simulink model "PRH_PI"  (R2021a)
settings: Solver=FixedStepDiscrete  StartTime=0.0  StopTime=4  RelTol=1e-3
values from neighbouring files (symbols this model uses):
  kp = place(A, B, [-8+.8i -8-.8i -9+.9i -9-.9i, -2+.1i, -2-.1i])    [HeightControlWithStableAngle.m]
  kr = transpose(transpose(V)*(V*transpose(V))^-1)    [HeightControlWithStableAngle.m]    (also in YawPitchRollHeightControl.m)
undefined symbols (not defined in the file or in its folder): DiscIntNeverNeededParam, Newton, Raphson
settings Model: Creator=tocay  LastModifiedBy=tocay
settings OptimizationCC: DefaultParameterBehavior=Inlined  UseDivisionForNetSlopeComputation=on  GainParamInheritBuiltInType=on  UseFloatMulNetSlope=on  InlineInvariantSignals=on  PassReuseOutputArgsAs=Individual arguments  ZeroExternalMemoryAtStartup=off  ZeroInternalMemoryAtStartup=off  NoFixptDivByZeroProtection=on  EfficientFloat2IntCast=on  LifeSpan=1  OptimizeBlockOrder=speed  DifferentSizesBufferReuse=on  EfficientTunableParamExpr=on
settings DebuggingCC: ParameterTunabilityLossMsg=error
settings HardwareCC: ProdBitPerInt=16  ProdBitPerPointer=8  ProdBitPerSizeT=24  ProdBitPerPtrDiffT=24  ProdLargestAtomicFloat=None  ProdWordSize=8  ProdLongLongMode=on  ProdHWDeviceType=Microchip->PIC18
settings SFSimCC: MATLABDynamicMemAlloc=off
settings RTWCC: SystemTargetFile=ert.tlc  GenCodeOnly=on  PackageName=PRH_at2.zip  TemplateMakefile=ert_default_tmf  TargetLang=C++
settings CodeAppCC: ForceParamTrailComments=on  IgnoreCustomStorageClasses=off  OperatorAnnotations=on  SimulinkDataObjDesc=on  SFDataObjDesc=on  CustomSymbolStrGlobalVar=rt$N$M  CustomSymbolStrType=$N$M  CustomSymbolStrFcn=$N$M$F  CustomSymbolStrMacro=$N$M  InsertBlockDesc=on
settings ERTTargetCC: TargetLangStandard=C++03 (ISO)  GenerateSampleERTMain=on  IncludeMdlTerminateFcn=off  CombineSignalStateStructs=on  SuppressErrorStatus=on  SupportAbsoluteTime=off  CodeInterfacePackaging=C++ class  SupportComplex=off  InlinedParameterPlacement=NonHierarchical  RootIOFormat=Structure reference  ERTCustomFileTemplate=example_file_process.tlc  ERTFilePackagingFormat=CompactWithDataFile

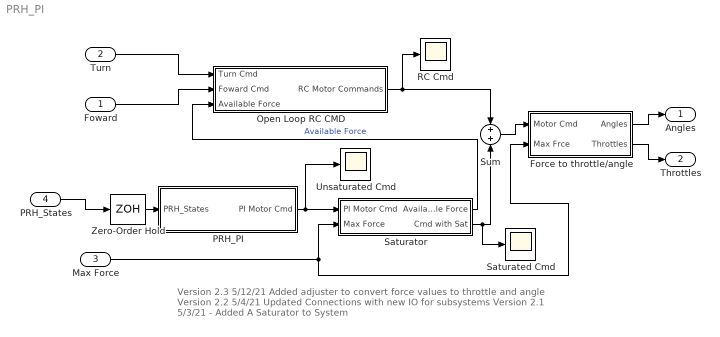
== system PRH_PI ==
  note: Version 2.3 5/12/21 Added adjuster to convert force values to throttle and angle
      | Version 2.2 5/4/21 Updated Connections with new IO for subsystems
      | Version 2.1 5/3/21 - Added A Saturator to System
  Foward : Inport
  Turn : Inport  Port=2
  Max Force : Inport  Port=3
  PRH_States : Inport  Port=4
  Force to throttle/angle : Subsystem
  Open Loop RC CMD : Subsystem
  PRH_PI : Subsystem
  RC Cmd : Scope
  Saturated Cmd : Scope
  Saturator : Subsystem
  Sum : Sum
  Unsaturated Cmd : Scope
  Zero-Order Hold : ZeroOrderHold  SampleTime=-1
  Angles : Outport
  Throttles : Outport  Port=2
  wires:
  Turn/1 -> Open Loop RC CMD/1(Turn Cmd)
  Open Loop RC CMD/1(RC Motor Commands) -> RC Cmd/1, Sum/1
  PRH_PI/1(PI Motor Cmd) -> Unsaturated Cmd/1, Saturator/1(PI Motor Cmd)
  Sum/1 -> Force to throttle/angle/1(Motor Cmd)
  Force to throttle/angle/2(Throttles) -> Throttles/1
  Force to throttle/angle/1(Angles) -> Angles/1
  Foward/1 -> Open Loop RC CMD/2(Foward Cmd)
  Saturator/1(Available Force) -> Open Loop RC CMD/3(Available Force)  "Available Force"
  Saturator/2(Cmd with Sat) -> Saturated Cmd/1, Sum/2
  Max Force/1 -> Saturator/2(Max Force), Force to throttle/angle/2(Max Frce)
  Zero-Order Hold/1 -> PRH_PI/1(PRH_States)
  PRH_States/1 -> Zero-Order Hold/1

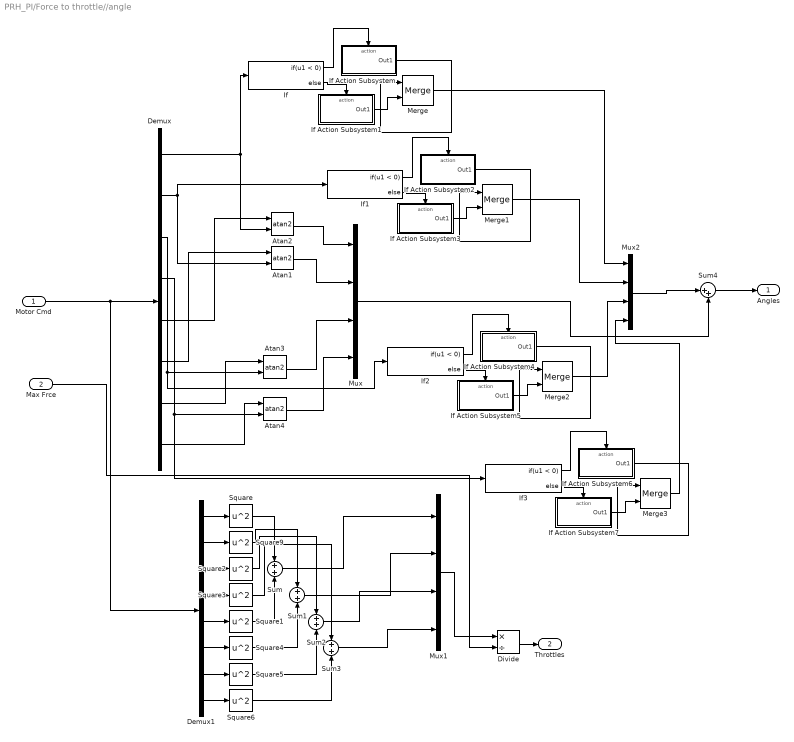
== system PRH_PI/Force to throttle//angle ==
  Motor Cmd : Inport
  Max Frce : Inport  Port=2
  Atan{1..4} (4 alike) : Trigonometry  Operator=atan2
  Demux : Demux  Outputs=8
  Demux1 : Demux  Outputs=8
  Divide : Product  Inputs=*/
  If{,1..3} (4 alike) : If  IfExpression=u1 < 0
  If Action Subsystem : Subsystem  TreatAsAtomicUnit=on
  If Action Subsystem1 : Subsystem  TreatAsAtomicUnit=on
  If Action Subsystem2 : Subsystem  TreatAsAtomicUnit=on
  If Action Subsystem3 : Subsystem  TreatAsAtomicUnit=on
  If Action Subsystem4 : Subsystem  TreatAsAtomicUnit=on
  If Action Subsystem5 : Subsystem  TreatAsAtomicUnit=on
  If Action Subsystem6 : Subsystem  TreatAsAtomicUnit=on
  If Action Subsystem7 : Subsystem  TreatAsAtomicUnit=on
  Merge{,1..3} (4 alike) : Merge
  Mux : Mux
  Mux1 : Mux
  Mux2 : Mux
  Square{,1..6,9} (8 alike) : Math  Operator=square  SaturateOnIntegerOverflow=on
  Sum{,1..3} (4 alike) : Sum
  Sum4 : Sum  Inputs=|++
  Angles : Outport
  Throttles : Outport  Port=2
  wires:
  Demux/5 -> Atan2/1
  Demux/1 -> Atan2/2, If/1
  Demux/6 -> Atan1/1
  Demux/7 -> Atan3/1
  Demux/8 -> Atan4/1
  Demux/4 -> If3/1, Atan4/2
  Demux/3 -> If2/1, Atan3/2
  Demux/2 -> Atan1/2, If1/1
  Atan2/1 -> Mux/1
  Atan1/1 -> Mux/2
  Atan3/1 -> Mux/3
  Atan4/1 -> Mux/4
  Square3/1 -> Sum3/1
  Square1/1 -> Sum/2
  Demux1/8 -> Square6/1
  Square/1 -> Sum/1
  Sum/1 -> Mux1/1
  Sum1/1 -> Mux1/2
  Demux1/7 -> Square5/1
  Square5/1 -> Sum2/2
  Square6/1 -> Sum3/2
  Sum2/1 -> Mux1/3
  Square2/1 -> Sum2/1
  Square4/1 -> Sum1/2
  Demux1/1 -> Square/1
  Demux1/6 -> Square4/1
  Demux1/5 -> Square1/1
  Demux1/3 -> Square2/1
  Demux1/2 -> Square9/1
  Square9/1 -> Sum1/1
  Motor Cmd/1 -> Demux1/1, Demux/1
  Demux1/4 -> Square3/1
  Sum3/1 -> Mux1/4
  Max Frce/1 -> Divide/2
  Mux1/1 -> Divide/1
  Divide/1 -> Throttles/1
  If/1 -> If Action Subsystem/Action
  If/2 -> If Action Subsystem1/Action
  If Action Subsystem/1(Out1) -> Merge/1
  If Action Subsystem1/1(Out1) -> Merge/2
  If Action Subsystem2/1(Out1) -> Merge1/1
  If Action Subsystem3/1(Out1) -> Merge1/2
  If1/2 -> If Action Subsystem3/Action
  If1/1 -> If Action Subsystem2/Action
  If Action Subsystem4/1(Out1) -> Merge2/1
  If Action Subsystem5/1(Out1) -> Merge2/2
  If2/2 -> If Action Subsystem5/Action
  If2/1 -> If Action Subsystem4/Action
  If Action Subsystem6/1(Out1) -> Merge3/1
  If Action Subsystem7/1(Out1) -> Merge3/2
  If3/2 -> If Action Subsystem7/Action
  If3/1 -> If Action Subsystem6/Action
  Merge/1 -> Mux2/1
  Merge1/1 -> Mux2/2
  Merge2/1 -> Mux2/3
  Merge3/1 -> Mux2/4
  Mux2/1 -> Sum4/1
  Mux/1 -> Sum4/2
  Sum4/1 -> Angles/1

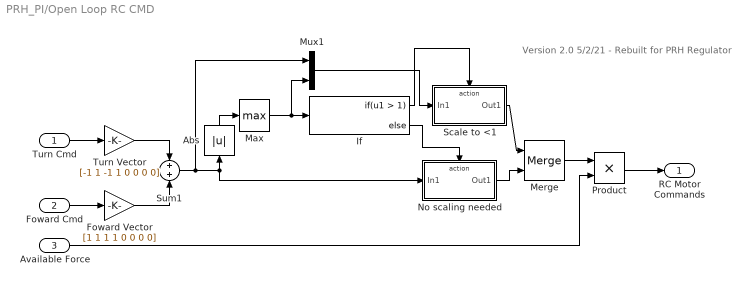
== system PRH_PI/Open Loop RC CMD ==
  note: Version 2.0 5/2/21 - Rebuilt for PRH Regulator
  Turn Cmd : Inport
  Foward Cmd : Inport  Port=2
  Available Force : Inport  Port=3
  Abs : Abs
  Foward Vector : Gain  Gain=[1 1 1 1 0 0 0 0]
  If : If  IfExpression=u1 > 1
  Max : MinMax  Function=max
  Merge : Merge
  Mux1 : Mux  Inputs=2
  No scaling needed : Subsystem  TreatAsAtomicUnit=on
  Product : Product
  Scale to <1 : Subsystem  TreatAsAtomicUnit=on
  Sum1 : Sum
  Turn Vector : Gain  Gain=[-1 1 -1 1 0 0 0 0]
  RC Motor Commands : Outport
  wires:
  Mux1/1 -> Scale to <1/1(In1)
  Sum1/1 -> Mux1/1, Abs/1, No scaling needed/1(In1)
  Scale to <1/1(Out1) -> Merge/1
  Foward Vector/1 -> Sum1/2
  If/2 -> No scaling needed/Action
  If/1 -> Scale to <1/Action
  Abs/1 -> Max/1
  Turn Cmd/1 -> Turn Vector/1
  Foward Cmd/1 -> Foward Vector/1
  Max/1 -> Mux1/2, If/1
  No scaling needed/1(Out1) -> Merge/2
  Turn Vector/1 -> Sum1/1
  Product/1 -> RC Motor Commands/1
  Merge/1 -> Product/1
  Available Force/1 -> Product/2

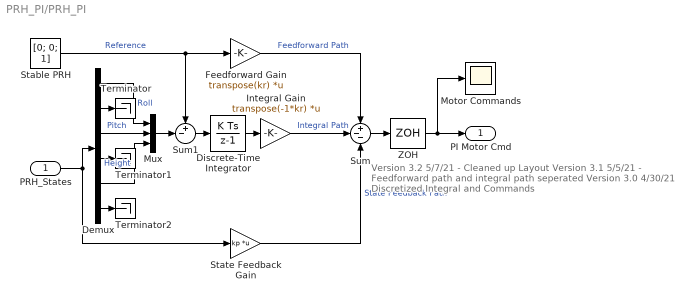
== system PRH_PI/PRH_PI ==
  note: Version 3.2 5/7/21 - Cleaned up Layout
      | Version 3.1 5/5/21 - Feedforward path and integral path seperated
      | Version 3.0 4/30/21 Discretized Integral and Commands
  PRH_States : Inport
  Demux : Demux  Outputs=6
  Discrete-Time Integrator : DiscreteIntegrator  SampleTime=-1  ICPrevOutput=DiscIntNeverNeededParam  ICPrevScaledInput=DiscIntNeverNeededParam
  Feedforward Gain : Gain  Gain=transpose(kr)  Multiplication=Matrix(K*u)
  Integral Gain : Gain  Gain=transpose(-1*kr)  Multiplication=Matrix(K*u)
  Motor Commands : Scope
  Mux : Mux  Inputs=3
  Stable PRH : Constant  Value=[0; 0; 1]  VectorParams1D=off
  State Feedback Gain : Gain  Gain=kp  Multiplication=Matrix(K*u)
  Sum : Sum  Inputs=+--
  Sum1 : Sum  Inputs=+-|
  Terminator : Terminator
  Terminator1 : Terminator
  Terminator2 : Terminator
  ZOH : ZeroOrderHold  SampleTime=-1
  PI Motor Cmd : Outport
  wires:
  Discrete-Time Integrator/1 -> Integral Gain/1
  Feedforward Gain/1 -> Sum/1  "Feedforward Path"
  Demux/6 -> Terminator2/1
  Demux/3 -> Mux/2  "Pitch"
  State Feedback Gain/1 -> Sum/3  "State Feedback Path"
  Stable PRH/1 -> Sum1/1, Feedforward Gain/1  "Reference"
  Demux/1 -> Mux/1  "Roll"
  Sum1/1 -> Discrete-Time Integrator/1
  Demux/2 -> Terminator/1
  Demux/4 -> Terminator1/1
  Integral Gain/1 -> Sum/2  "Integral Path"
  PRH_States/1 -> State Feedback Gain/1, Demux/1
  Demux/5 -> Mux/3  "Height"
  Sum/1 -> ZOH/1
  ZOH/1 -> PI Motor Cmd/1, Motor Commands/1
  Mux/1 -> Sum1/2

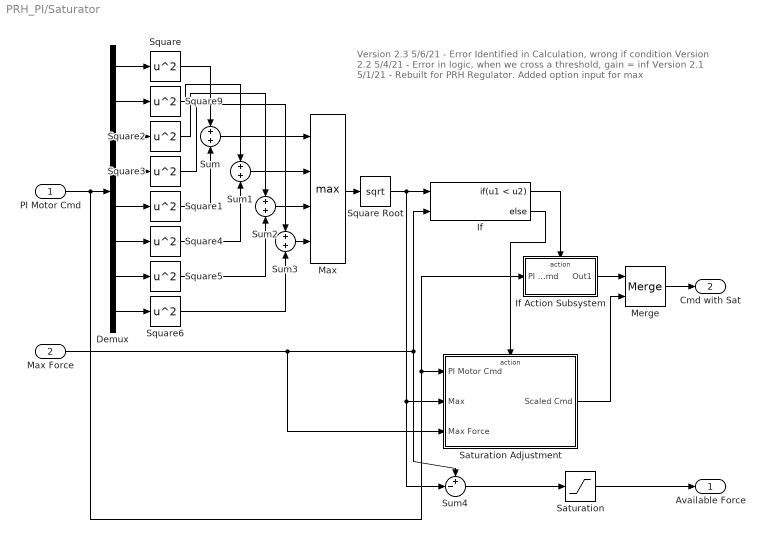
== system PRH_PI/Saturator ==
  note: Version 2.3 5/6/21 - Error Identified in Calculation, wrong if condition
      | Version 2.2 5/4/21 - Error in logic, when we cross a threshold, gain = inf
      | Version 2.1 5/1/21 - Rebuilt for PRH Regulator. Added option input for max
  PI Motor Cmd : Inport
  Max Force : Inport  Port=2
  Demux : Demux  Outputs=8
  If : If  NumInputs=2  IfExpression=u1 < u2
  If Action Subsystem : Subsystem  TreatAsAtomicUnit=on
  Max : MinMax  Function=max  Inputs=4
  Merge : Merge
  Saturation : Saturate  UpperLimit=5  LowerLimit=0
  Saturation Adjustment : Subsystem  TreatAsAtomicUnit=on
  Square{,1..6,9} (8 alike) : Math  Operator=square  SaturateOnIntegerOverflow=on
  Square Root : Sqrt  OutputSignalType=real  AlgorithmType=Newton-Raphson  SaturateOnIntegerOverflow=on
  Sum{,1..3} (4 alike) : Sum
  Sum4 : Sum  Inputs=+-|
  Available Force : Outport
  Cmd with Sat : Outport  Port=2
  wires:
  PI Motor Cmd/1 -> Saturation Adjustment/1(PI Motor Cmd), If Action Subsystem/1(PI Motor Cmd), Demux/1
  Demux/1 -> Square/1
  Demux/5 -> Square1/1
  Demux/2 -> Square9/1
  Demux/3 -> Square2/1
  Demux/4 -> Square3/1
  Demux/6 -> Square4/1
  Square/1 -> Sum/1
  Square9/1 -> Sum1/1
  Square4/1 -> Sum1/2
  Square2/1 -> Sum2/1
  Sum/1 -> Max/1
  Sum1/1 -> Max/2
  Sum2/1 -> Max/3
  Max Force/1 -> Saturation Adjustment/3(Max Force), Sum4/1, If/2
  If/1 -> If Action Subsystem/Action
  If/2 -> Saturation Adjustment/Action
  Saturation Adjustment/1(Scaled Cmd) -> Merge/2
  If Action Subsystem/1(Out1) -> Merge/1
  Merge/1 -> Cmd with Sat/1
  Sum4/1 -> Saturation/1
  Saturation/1 -> Available Force/1
  Demux/7 -> Square5/1
  Demux/8 -> Square6/1
  Square1/1 -> Sum/2
  Square5/1 -> Sum2/2
  Square6/1 -> Sum3/2
  Square3/1 -> Sum3/1
  Sum3/1 -> Max/4
  Max/1 -> Square Root/1
  Square Root/1 -> Sum4/2, Saturation Adjustment/2(Max), If/1

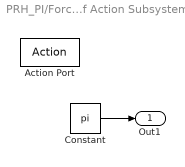
== system PRH_PI/Force to throttle//angle/If Action Subsystem ==
  Action Port : ActionPort  ActionPortLabel=if(u1 < 0)
  Constant : Constant  Value=pi
  Out1 : Outport
  wires:
  Constant/1 -> Out1/1

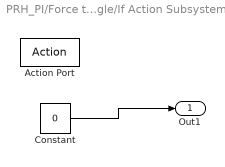
== system PRH_PI/Force to throttle//angle/If Action Subsystem1 ==
  Action Port : ActionPort  ActionPortLabel=else
  Constant : Constant  Value=0
  Out1 : Outport
  wires:
  Constant/1 -> Out1/1

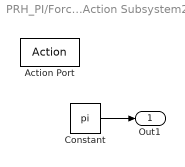
== system PRH_PI/Force to throttle//angle/If Action Subsystem2 ==
  Action Port : ActionPort  ActionPortLabel=if(u1 < 0)
  Constant : Constant  Value=pi
  Out1 : Outport
  wires:
  Constant/1 -> Out1/1

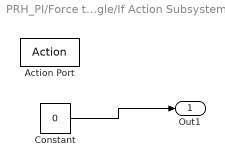
== system PRH_PI/Force to throttle//angle/If Action Subsystem3 ==
  Action Port : ActionPort  ActionPortLabel=else
  Constant : Constant  Value=0
  Out1 : Outport
  wires:
  Constant/1 -> Out1/1

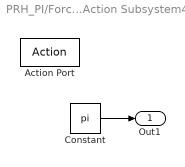
== system PRH_PI/Force to throttle//angle/If Action Subsystem4 ==
  Action Port : ActionPort  ActionPortLabel=if(u1 < 0)
  Constant : Constant  Value=pi
  Out1 : Outport
  wires:
  Constant/1 -> Out1/1

== system PRH_PI/Force to throttle//angle/If Action Subsystem5 ==
  Action Port : ActionPort  ActionPortLabel=else
  Constant : Constant  Value=0
  Out1 : Outport
  wires:
  Constant/1 -> Out1/1

== system PRH_PI/Force to throttle//angle/If Action Subsystem6 ==
  Action Port : ActionPort  ActionPortLabel=if(u1 < 0)
  Constant : Constant  Value=pi
  Out1 : Outport
  wires:
  Constant/1 -> Out1/1

== system PRH_PI/Force to throttle//angle/If Action Subsystem7 ==
  Action Port : ActionPort  ActionPortLabel=else
  Constant : Constant  Value=0
  Out1 : Outport
  wires:
  Constant/1 -> Out1/1

== system PRH_PI/Open Loop RC CMD/No scaling needed ==
  In1 : Inport
  Action Port : ActionPort  ActionPortLabel=else
  Out1 : Outport
  wires:
  In1/1 -> Out1/1

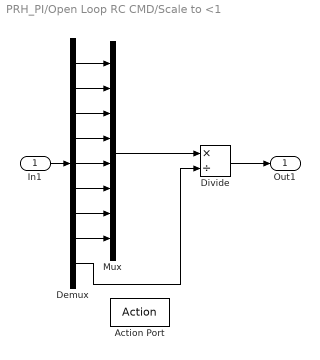
== system PRH_PI/Open Loop RC CMD/Scale to <1 ==
  In1 : Inport
  Action Port : ActionPort  ActionPortLabel=if(u1 > 1)
  Demux : Demux  Outputs=9
  Divide : Product  Inputs=*/
  Mux : Mux  Inputs=8
  Out1 : Outport
  wires:
  In1/1 -> Demux/1
  Demux/1 -> Mux/1
  Demux/2 -> Mux/2
  Demux/3 -> Mux/3
  Demux/5 -> Mux/5
  Demux/4 -> Mux/4
  Demux/6 -> Mux/6
  Demux/7 -> Mux/7
  Demux/8 -> Mux/8
  Mux/1 -> Divide/1
  Demux/9 -> Divide/2
  Divide/1 -> Out1/1

== system PRH_PI/Saturator/If Action Subsystem ==
  PI Motor Cmd : Inport
  Action Port : ActionPort  ActionPortLabel=if(u1 < u2)
  Out1 : Outport
  wires:
  PI Motor Cmd/1 -> Out1/1

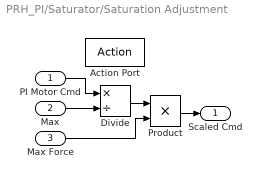
== system PRH_PI/Saturator/Saturation Adjustment ==
  PI Motor Cmd : Inport
  Max : Inport  Port=2
  Max Force : Inport  Port=3
  Action Port : ActionPort  ActionPortLabel=else
  Divide : Product  Inputs=*/
  Product : Product
  Scaled Cmd : Outport
  wires:
  PI Motor Cmd/1 -> Divide/1
  Divide/1 -> Product/1
  Max Force/1 -> Product/2
  Product/1 -> Scaled Cmd/1
  Max/1 -> Divide/2
